simulink model "model_mit"  (R2022b)
settings: Solver=ode45  StartTime=0.0  StopTime=tsim  RelTol=1e-3
values from neighbouring files (symbols this model uses):
  A = [-0.0125,  0.0126,  0.0000 ... (first row only)    [main.m]
  am = 0.008    [main.m]
  B = [-0.0091 ... (first row only)    [main.m]
  bm = 0.008    [main.m]
  C = [0.0, 0.0, 1.0]    [main.m]
  gamma_f = 0.05    [main.m]
  gamma_q = 0.06    [main.m]
  Kos3 = 9.0000    (= 9)    [main.m]
  Ks2 = -27.5827    [main.m]
  ref_ss = x3_ss    (= 4.8098)    [main.m]
  sigma = 0.00005    (= 5e-05)    [main.m]
  sign_b = -1    [main.m]
  t1 = 40000    [main.m]
  u1_ss = -4    [main.m]
  u_max = 10    [main.m]
  u_min = -10    [main.m]
  x3_ss = 4.8098    [main.m]
libraries: simulink x1, spsStairGeneratorLib x1
settings Model: Creator=krist  LastModifiedBy=krist
settings DebuggingCC: UnconnectedInputMsg=warning  UnconnectedOutputMsg=warning  UnconnectedLineMsg=warning
settings ModelReferenceCC: EnableRefExpFcnMdlSchedulingChecks=on
settings RTWCC: DLArmComputeVersion=19.05

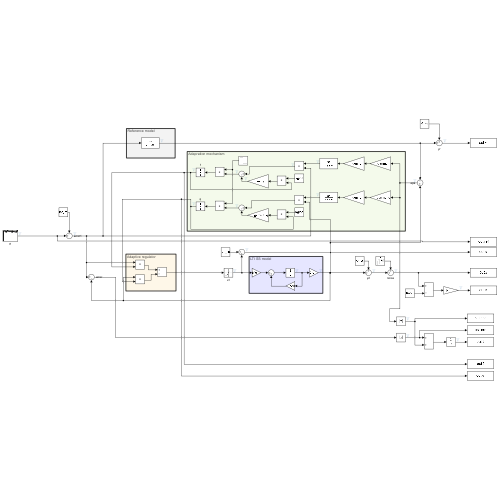
[thumbnail: Simulink's stored preview of the top-level diagram]
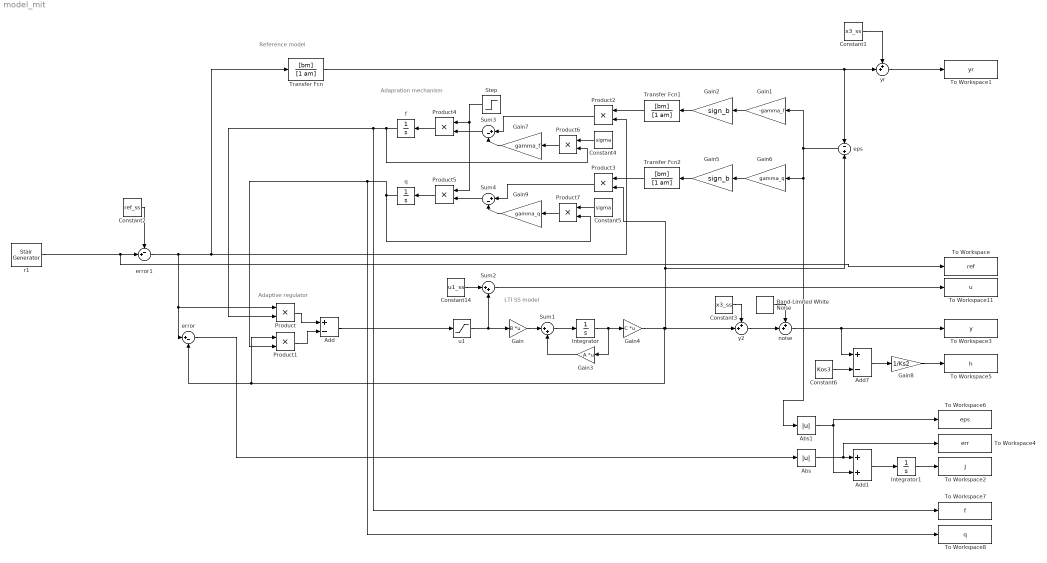
== system model_mit ==
  note: LTI SS model
  note: Adaptive regulator
  note: Adapration mechanism
  note: Reference model
  Abs : Abs  SaturateOnIntegerOverflow=off
  Abs1 : Abs  SaturateOnIntegerOverflow=off
  Add : Sum  Inputs=+-
  Add1 : Sum
  Add7 : Sum  Inputs=+-
  Band-Limited White Noise : simulink/Sources/Band-Limited White Noise  Cov=5*10^-7  Ts=0.1  seed=[23341]
  Constant1 : Constant  Value=x3_ss
  Constant14 : Constant  Value=u1_ss
  Constant2 : Constant  Value=ref_ss
  Constant3 : Constant  Value=x3_ss
  Constant4 : Constant  Value=sigma
  Constant5 : Constant  Value=sigma
  Constant6 : Constant  Value=Kos3
  Gain : Gain  Gain=B  Multiplication=Matrix(K*u)
  Gain1 : Gain  Gain=-gamma_f
  Gain2 : Gain  Gain=sign_b
  Gain3 : Gain  Gain=A  Multiplication=Matrix(K*u)
  Gain4 : Gain  Gain=C  Multiplication=Matrix(K*u)
  Gain5 : Gain  Gain=sign_b
  Gain6 : Gain  Gain=gamma_q
  Gain7 : Gain  Gain=gamma_f
  Gain8 : Gain  Gain=1/Ks2
  Gain9 : Gain  Gain=gamma_q
  Integrator : Integrator
  Integrator1 : Integrator
  Product{,1..7} (8 alike) : Product
  Step : Step  Time=t1  Before=1  After=0  SampleTime=0
  Sum1 : Sum  Inputs=|++
  Sum2 : Sum  Inputs=|++
  Sum3 : Sum  Inputs=|+-
  Sum4 : Sum  Inputs=|+-
  To Workspace : ToWorkspace  VariableName=ref  SaveFormat=Timeseries  SampleTime=-1
  To Workspace1 : ToWorkspace  VariableName=yr  SaveFormat=Timeseries  SampleTime=-1
  To Workspace11 : ToWorkspace  VariableName=u  SaveFormat=Timeseries  SampleTime=-1
  To Workspace2 : ToWorkspace  VariableName=J  SaveFormat=Timeseries  SampleTime=-1
  To Workspace3 : ToWorkspace  VariableName=y  SaveFormat=Timeseries  SampleTime=-1
  To Workspace4 : ToWorkspace  VariableName=err  SaveFormat=Timeseries  SampleTime=-1
  To Workspace5 : ToWorkspace  VariableName=h  SaveFormat=Timeseries  SampleTime=-1
  To Workspace6 : ToWorkspace  VariableName=eps  SaveFormat=Timeseries  SampleTime=-1
  To Workspace7 : ToWorkspace  VariableName=f  SaveFormat=Timeseries  SampleTime=-1
  To Workspace8 : ToWorkspace  VariableName=q  SaveFormat=Timeseries  SampleTime=-1
  Transfer Fcn : TransferFcn  Numerator=[bm]  Denominator=[1 am]
  Transfer Fcn1 : TransferFcn  Numerator=[bm]  Denominator=[1 am]
  Transfer Fcn2 : TransferFcn  Numerator=[bm]  Denominator=[1 am]
  eps : Sum  Inputs=-|+
  error : Sum  Inputs=|+-
  error1 : Sum  Inputs=-+|
  f : Integrator
  noise : Sum  Inputs=++|
  q : Integrator
  r1 : spsStairGeneratorLib/Stair Generator  t=ref_in.Times  e=ref_in.Vals  Ts=0
  u1 : Saturate  UpperLimit=u_max-u1_ss  LowerLimit=u_min-u1_ss
  y2 : Sum  Inputs=++|
  yr : Sum  Inputs=++|
  wires:
  r1/1 -> To Workspace/1, error1/2
  Constant3/1 -> y2/1
  Add7/1 -> Gain8/1
  Constant6/1 -> Add7/2
  u1/1 -> Sum2/2, Gain/1
  Gain/1 -> Sum1/1
  Sum1/1 -> Integrator/1
  Gain3/1 -> Sum1/2
  Integrator/1 -> Gain3/1, Gain4/1
  Sum2/1 -> To Workspace11/1
  Gain4/1 -> eps/2, Product3/2, y2/2, Product1/1, error/2
  Constant14/1 -> Sum2/1
  Add/1 -> u1/1
  error/1 -> Abs/1
  Gain8/1 -> To Workspace5/1
  Add1/1 -> Integrator1/1
  Integrator1/1 -> To Workspace2/1
  Abs/1 -> Add1/1, To Workspace4/1
  Abs1/1 -> Add1/2, To Workspace6/1
  y2/1 -> noise/2
  noise/1 -> Add7/1, To Workspace3/1
  Band-Limited White Noise/1 -> noise/1
  Product/1 -> Add/1
  Product1/1 -> Add/2
  f/1 -> Product6/2, To Workspace7/1, Product/2
  q/1 -> To Workspace8/1, Product1/2, Product7/2
  Transfer Fcn/1 -> yr/2, eps/1
  eps/1 -> Abs1/1, Gain6/1, Gain1/1
  Gain1/1 -> Gain2/1
  Gain2/1 -> Transfer Fcn1/1
  Transfer Fcn1/1 -> Product2/1
  Transfer Fcn2/1 -> Product3/1
  Gain5/1 -> Transfer Fcn2/1
  Gain6/1 -> Gain5/1
  Product4/1 -> f/1
  Product5/1 -> q/1
  Step/1 -> Product4/1, Product5/1
  Product2/1 -> Sum3/1
  Sum3/1 -> Product4/2
  Constant4/1 -> Product6/1
  Gain7/1 -> Sum3/2
  Product6/1 -> Gain7/1
  Gain9/1 -> Sum4/2
  Product7/1 -> Gain9/1
  Constant5/1 -> Product7/1
  Sum4/1 -> Product5/2
  Product3/1 -> Sum4/1
  yr/1 -> To Workspace1/1
  Constant1/1 -> yr/1
  Constant2/1 -> error1/1
  error1/1 -> Product/1, error/1, Transfer Fcn/1, Product2/2
